simulink subsystem "CAN"  (R2022b)
settings: Solver=VariableStepAuto  StartTime=0.0  StopTime=10.0  RelTol=1e-3
settings Model: Creator=serga  LastModifiedBy=serga

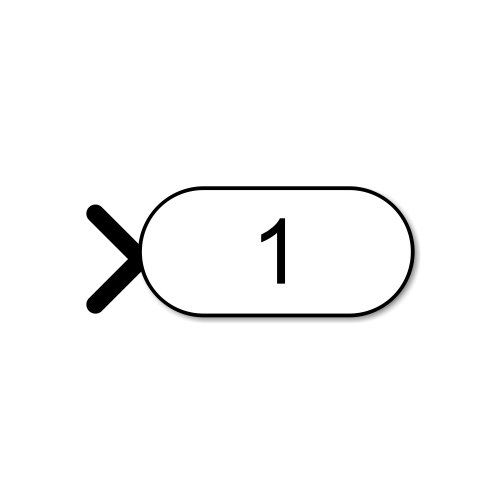
[thumbnail: Simulink's stored preview of the top-level diagram]
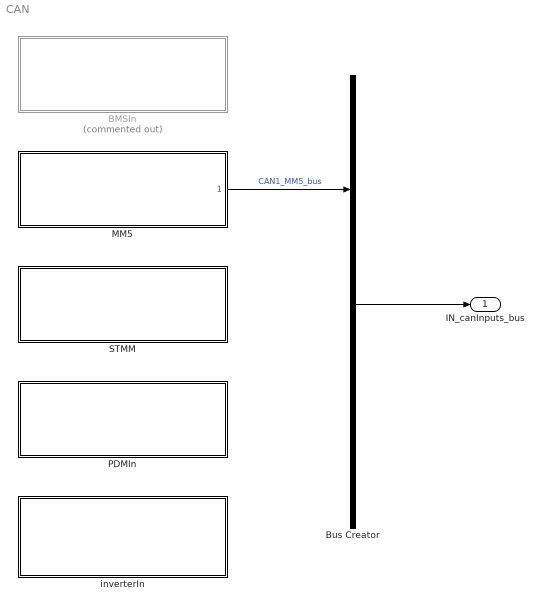
== system CAN ==
  BMSIn : Subsystem  Commented=on  ReferencedSubsystem=BMSIn
  Bus Creator : BusCreator  Inputs=2
  MM5 : Subsystem  ReferencedSubsystem=MM5
  PDMIn : Subsystem  ReferencedSubsystem=PDMIn
  STMM : Subsystem  ReferencedSubsystem=STMM
  inverterIn : Subsystem  ReferencedSubsystem=inverterIn
  IN_canInputs_bus : Outport
  wires:
  MM5/1 -> Bus Creator/1  "CAN1_MM5_bus"
  Bus Creator/1 -> IN_canInputs_bus/1
